simulink model "Jacinv"  (R2019b)
settings: Solver=VariableStepAuto  StartTime=0.0  StopTime=4  RelTol=1e-3
undefined symbols (not defined in the file or in its folder): DiscIntNeverNeededParam, q0, Tc
settings Model: Creator=GA  LastModifiedBy=GA

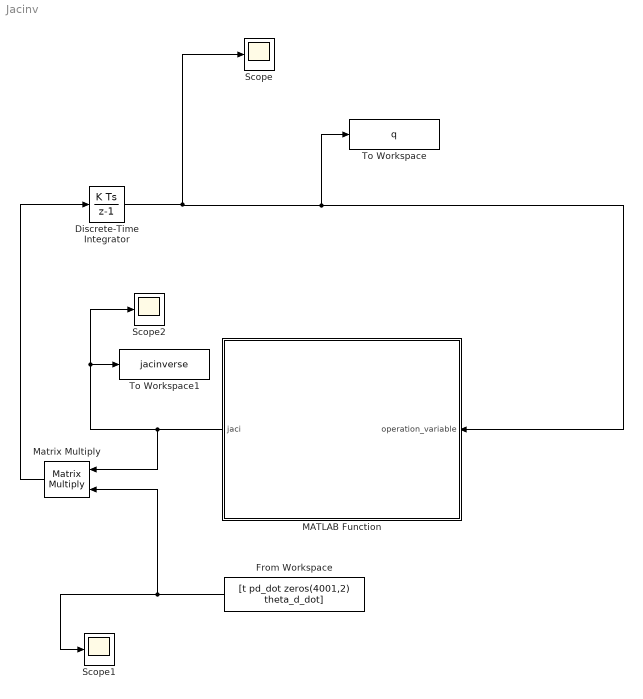
== system Jacinv ==
  Discrete-Time Integrator : DiscreteIntegrator  InitialCondition=q0  SampleTime=-1  ICPrevOutput=DiscIntNeverNeededParam  ICPrevScaledInput=DiscIntNeverNeededParam
  From Workspace : FromWorkspace  VariableName=[t pd_dot zeros(4001,2) theta_d_dot]  SampleTime=Tc
  MATLAB Function : MATLAB Function  TreatAsAtomicUnit=on
  Matrix Multiply : Product  Multiplication=Matrix(*)
  Scope : Scope
  Scope1 : Scope
  Scope2 : Scope
  To Workspace : ToWorkspace  VariableName=q  SaveFormat=Timeseries  SampleTime=-1
  To Workspace1 : ToWorkspace  VariableName=jacinverse  SaveFormat=Timeseries  SampleTime=-1
  wires:
  Discrete-Time Integrator/1 -> Scope/1, To Workspace/1, MATLAB Function/1(operation_variable)
  MATLAB Function/1(jaci) -> Scope2/1, To Workspace1/1, Matrix Multiply/1
  From Workspace/1 -> Scope1/1, Matrix Multiply/2
  Matrix Multiply/1 -> Discrete-Time Integrator/1

== matlab function Jacinv/MATLAB Function ==
  data: operation_variable input; jaci output
function jaci = jacobians(operation_variable)
d0 = 1;
a1 = 0.5;
a2 = 0.5;

jac = zeros(6,4);
jac(1,1) =	-a1*sin(operation_variable(1))-a2*sin(operation_variable(1)+operation_variable(2));
jac(1,2) = -a2*sin(operation_variable(1)+operation_variable(2));
jac(2,1) = a1*cos(operation_variable(1))+a2*cos(operation_variable(1)+operation_variable(2));
jac(2,2) = a2*cos(operation_variable(1)+operation_variable(2));
jac(3,3) = -1;
jac(6,1) = 1;
jac(6,2) = 1;
jac(6,4) = -1;

jaci = pinv(jac);
